simulink library "Feeder1_lib"  (Simulink 8.1)
settings: Solver=ode45  StartTime=0.0  StopTime=10.0  RelTol=1e-3
undefined symbols (not defined in the file): Left, Ts, type, V
libraries: breaker_lib x16, cables_lib x15, transformer_lib x9, Load_lib x6, ssn_lib x6, fault_lib x3, rtlab x2, powerlib x1, HWController_Diesel_GenSet_4MVA_lib x1, Motor_InductionMachine_lib x1, PQFV_lib x1
settings Model: Creator=re25624  LastModifiedBy=RE25624

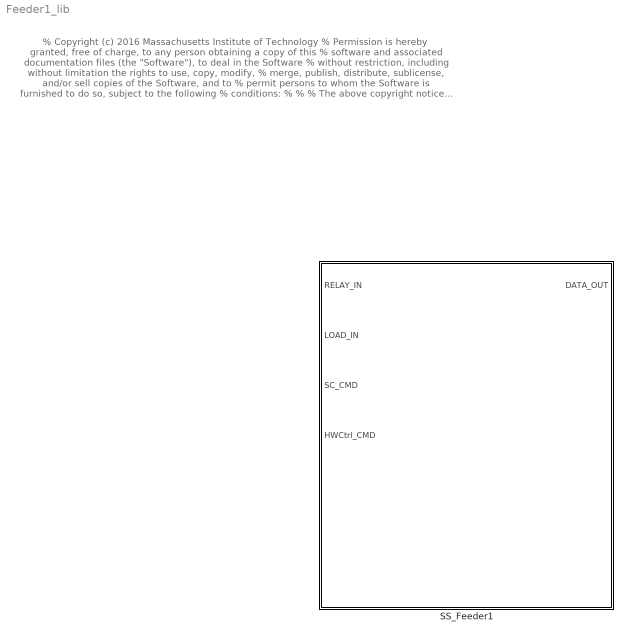
== system Feeder1_lib ==
  note: % Copyright (c) 2016 Massachusetts Institute of Technology
      | % Permission is hereby granted, free of charge, to any person obtaining a copy of this
      | % software and associated documentation files (the "Software"), to deal in the Software
      | % without restriction, including without limitation the rights to use, copy, modify,
      | % merge, publish, distribute, sublicense, and/or sell copies of the Software, and to
      | % permit persons to whom the Software is furnished to do so, subject to the following
      | % conditions:
      | %
      | %
      | % The above copyright notice and this permission notice shall be included in
      | % all copies or substantial portions of the Software.
      | %
      | % THE SOFTWARE IS PROVIDED "AS IS", WITHOUT WARRANTY OF ANY KIND, EXPRESS OR IMPLIED,
      | % INCLUDING BUT NOT LIMITED TO THE WARRANTIES OF MERCHANTABILITY, FITNESS FOR A
      | % PARTICULAR PURPOSE AND NONINFRINGEMENT. IN NO EVENT SHALL THE AUTHORS OR COPYRIGHT
      | % HOLDERS BE LIABLE FOR ANY CLAIM, DAMAGES OR OTHER LIABILITY, WHETHER IN AN ACTION
      | % OF CONTRACT, TORT OR OTHERWISE, ARISING FROM, OUT OF OR IN CONNECTION WITH THE
      | % SOFTWARE OR THE USE OR OTHER DEALINGS IN THE SOFTWARE.
      | %
      | %
      | %%
  SS_Feeder1 : Subsystem

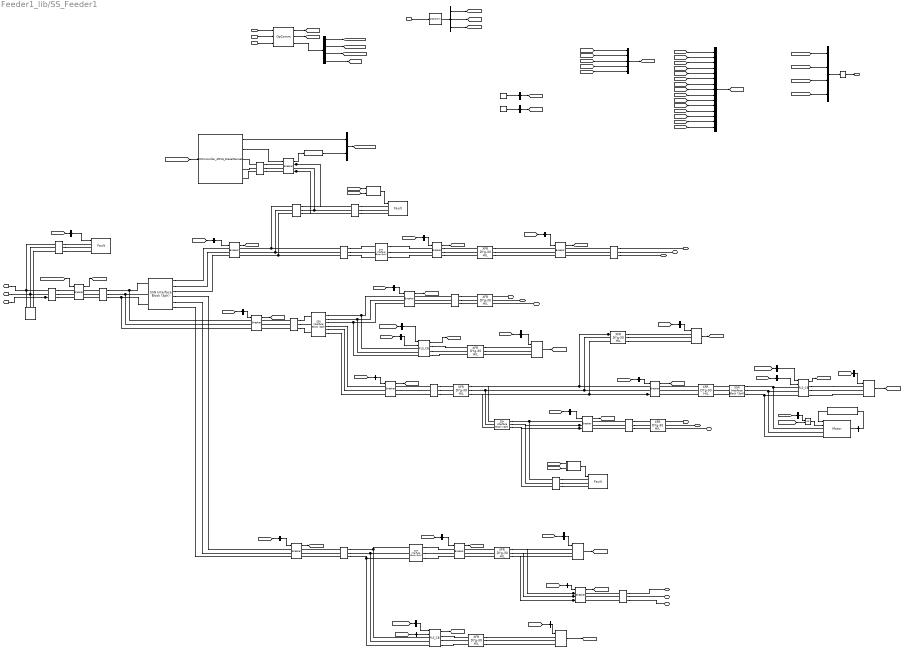
== system Feeder1_lib/SS_Feeder1 ==
  note: % Copyright (c) 2016 Massachusetts Institute of Technology
      | % Permission is hereby granted, free of charge, to any person obtaining a copy of this
      | % software and associated documentation files (the "Software"), to deal in the Software
      | % without restriction, including without limitation the rights to use, copy, modify,
      | % merge, publish, distribute, sublicense, and/or sell copies of the Software, and to
      | % permit persons to whom the Software is furnished to do so, subject to the following
      | % conditions:
      | %
      | %
      | % The above copyright notice and this permission notice shall be included in
      | % all copies or substantial portions of the Software.
      | %
      | % THE SOFTWARE IS PROVIDED "AS IS", WITHOUT WARRANTY OF ANY KIND, EXPRESS OR IMPLIED,
      | % INCLUDING BUT NOT LIMITED TO THE WARRANTIES OF MERCHANTABILITY, FITNESS FOR A
      | % PARTICULAR PURPOSE AND NONINFRINGEMENT. IN NO EVENT SHALL THE AUTHORS OR COPYRIGHT
      | % HOLDERS BE LIABLE FOR ANY CLAIM, DAMAGES OR OTHER LIABILITY, WHETHER IN AN ACTION
      | % OF CONTRACT, TORT OR OTHERWISE, ARISING FROM, OUT OF OR IN CONNECTION WITH THE
      | % SOFTWARE OR THE USE OR OTHER DEALINGS IN THE SOFTWARE.
      | %
      | %
      | %%
  note: connect to F3
  note: connect to F2
  note: connect to F2
  note: connect to F2
  RELAY_IN : Inport
  LOAD_IN : Inport  Port=2
  SC_CMD : Inport  Port=3
  HWCtrl_CMD : Inport  Port=4
  200 HP chiller compressor : Load_lib/200 HP chiller compressor
  2000 kVA4 : transformer_lib/XFR DYg-30 HIL  Rating=2000  Vp=4160  Vs=480  Z=5.75  XR=5.7
  2000 kVA5 : transformer_lib/XFR DYg-30 HIL  Rating=2000  Vp=4160  Vs=480  Z=5.75  XR=5.7
  2500 kVA : transformer_lib/XFR DYg-30 HIL  Rating=2500  Vp=13800  Vs=480  Z=5.75  XR=6.6
  2500 kVA2 : transformer_lib/XFR DYg-30 HIL  Rating=2500  Vp=13800  Vs=480  Z=5.56  XR=5.52
  3750 kVA1 : transformer_lib/XFR DYg-30 HIL  Rating=3750  Vp=13800  Vs=4160  Z=4.75  XR=11.4
  4/0AWG-Mutual1 : cables_lib/4//0AWG-Mutual  length=100  par_sets=1  ratio=3
  448 kvar inductor at 13.8kV  to cancel kvar produced by the stublines1 : powerlib/Elements/Three-Phase Parallel RLC Load  LConnTagsString=A|B|C  Configuration=Y (grounded)  NominalVoltage=13800  NominalFrequency=60  ActivePower=0  InductivePower=448e3  CapacitivePower=0  Measurements=None  LoadType=constant Z
  500 kVA2 : transformer_lib/XFR DYg-30 HIL  Rating=500  Vp=13800  Vs=480  Z=5  XR=4.9
  500 kVA3 : transformer_lib/XFR DYg-30 HIL  Rating=500  Vp=13800  Vs=208  Z=5  XR=4.9
  500kcmil-Mutual1 : cables_lib/500kcmil-Mutual  length=1000  par_sets=1  ratio=3
  500kcmil-Mutual2 : cables_lib/500kcmil-Mutual  length=10  par_sets=1  ratio=3
  500kcmil-Mutual3 : cables_lib/500kcmil-Mutual  length=10  par_sets=1  ratio=3
  500kcmil-Mutual4 : cables_lib/500kcmil-Mutual  length=10  par_sets=1  ratio=3
  500kcmil-Mutual9 : cables_lib/500kcmil-Mutual  length=100  par_sets=1  ratio=3
  Bus Creator : BusCreator  Inputs=1
  Bus Creator1 : BusCreator  Inputs=1
  Bus Creator2 : BusCreator
  Bus Creator3 : BusCreator  Inputs=5
  Bus Creator5 : BusCreator  Inputs=15
  Bus Creator6 : BusCreator  Inputs=2
  Bus Selector : BusSelector  OutputSignals=motor_1
  Bus Selector1 : BusSelector  OutputSignals=F1_CB_12
  Bus Selector10 : BusSelector  OutputSignals=F1_CB_2
  Bus Selector11 : BusSelector  OutputSignals=F1_CB_1
  Bus Selector12 : BusSelector  OutputSignals=F1_CB_5
  Bus Selector13 : BusSelector  OutputSignals=F1_CB_3
  Bus Selector14 : BusSelector  OutputSignals=F1_CB_6
  Bus Selector15 : BusSelector  OutputSignals=F1_CB_7
  Bus Selector16 : BusSelector  OutputSignals=F1_CB_10
  Bus Selector17 : BusSelector  OutputSignals=F1_CB_11
  Bus Selector18 : BusSelector  OutputSignals=F1_CB_9
  Bus Selector19 : BusSelector  OutputSignals=F1_CB_14
  Bus Selector2 : BusSelector  OutputSignals=F1_CB_4
  Bus Selector20 : BusSelector  OutputSignals=fault_cmd,motor_ONOFF.F1_motor_ONOFF,GridStatusCtrl.Grid_F1.Logic_trip
  Bus Selector21 : BusSelector  OutputSignals=HWCtrl.Diesel_Gen2,HWCtrl.SEL751_LogicTrip.F1.Logic_trip,HWCtrl.SEL2440_FLS,TestSeq
  Bus Selector22 : BusSelector  OutputSignals=RPM
  Bus Selector23 : BusSelector  OutputSignals=CB107
  Bus Selector24 : BusSelector  OutputSignals=CB104
  Bus Selector25 : BusSelector  OutputSignals=CB114
  Bus Selector26 : BusSelector  OutputSignals=fault_location_6
  Bus Selector3 : BusSelector  OutputSignals=I2
  Bus Selector4 : BusSelector  OutputSignals=C2
  Bus Selector5 : BusSelector  OutputSignals=P1
  Bus Selector6 : BusSelector  OutputSignals=C1
  Bus Selector7 : BusSelector  OutputSignals=I1
  Bus Selector8 : BusSelector  OutputSignals=F1_CB_13
  Bus Selector9 : BusSelector  OutputSignals=F1_CB_8
  C1 : cables_lib/500kcmil-Mutual  length=10  par_sets=1  ratio=3
  C101 : cables_lib/500kcmil-Mutual  length=1800  par_sets=1  ratio=3
  C102 : cables_lib/500kcmil-Mutual  length=5500  par_sets=1  ratio=3
  C103 : cables_lib/4//0AWG-Mutual  length=1000  par_sets=1  ratio=3
  C104 : cables_lib/500kcmil-Mutual  length=3000  par_sets=1  ratio=3
  C106 : cables_lib/500kcmil-Mutual  length=1500  par_sets=1  ratio=3
  C108 : cables_lib/500kcmil-Mutual  length=10  par_sets=1  ratio=3
  C109 : cables_lib/500kcmil-Mutual  length=1  par_sets=1  ratio=3
  C2 : cables_lib/500kcmil-Mutual  length=10  par_sets=1  ratio=3
  CB closed : Constant
  CB open : Constant  Value=0
  Critical_1 : Load_lib/Dynamic_Load  V=480  kVA=1200  PF=0.9  Ts=Ts
  Critical_2 : Load_lib/Dynamic_Load  V=480  kVA=1500  PF=0.9  Ts=Ts
  F1-GCB : breaker_lib/Breaker  Ts=Ts  mech_delay=cb_mech_delay
  F1_CB_{1..3,5..6,8..13} (11 alike) : breaker_lib/Breaker  Ts=Ts  mech_delay=cb_mech_delay
  F1_CB_14 : breaker_lib/FLS_CB  Ts=Ts  mech_delay=cb_mech_delay
  F1_CB_4 : breaker_lib/FLS_CB  Ts=Ts  mech_delay=cb_mech_delay
  F1_CB_7 : breaker_lib/FLS_CB  Ts=Ts  mech_delay=cb_mech_delay
  F1_PCC : breaker_lib/Breaker  Ts=Ts  mech_delay=cb_mech_delay
  Fault_2 : fault_lib/Fault  FaultResistance=0.1  GroundResistance=1.73  SnubberResistance=1E6
  Fault_3 : fault_lib/Fault  FaultResistance=0.1  GroundResistance=1.73  SnubberResistance=1E6
  Fault_6 : fault_lib/Fault  FaultResistance=0.1  GroundResistance=0.01  SnubberResistance=1E6
  HWController_4MVA_DieselGenset : HWController_Diesel_GenSet_4MVA_lib/HWController_4MVA_DieselGenset
  Interruptible_1 : Load_lib/Dynamic_Load  V=480  kVA=300  PF=0.9  Ts=Ts
  Interruptible_2 : Load_lib/Dynamic_Load  V=208  kVA=250  PF=0.9  Ts=Ts
  Logical Operator : Logic  Operator=OR  AllPortsSameDT=off  OutDataTypeStr=boolean
  Low imp xfr to handle stubline : transformer_lib/XFR DYg-30 HIL  Rating=5000  Vp=13800  Vs=500  Z=0.1  XR=10
  Low imp xfr to handle stubline1 : transformer_lib/XFR DYg-30 HIL  Rating=5000  Vp=4160  Vs=500  Z=0.1  XR=10
  Memory : Memory
  Motor : Motor_InductionMachine_lib/Motor
  OpComm1 : rtlab/OpComm  nbport=3  groupe_acq=1  subsys_rate=0  st=0  Synchronization=on  Interpolation=on  Threshold=1.0  Missed_Data=off  Sim_Time=off  Samples=off  dynSigOut=off  from_console=0  warning_done=off  writeOpCommFile=off  Offset=off
  OpComm2 : rtlab/OpComm  nbport=1  groupe_acq=1  subsys_rate=0  st=0  Synchronization=on  Interpolation=on  Threshold=1.0  Missed_Data=off  Sim_Time=off  Samples=off  dynSigOut=off  from_console=1  warning_done=off  writeOpCommFile=off  Offset=off
  PQFV : PQFV_lib/PQFV  VRMSLL=13800  Ts=Ts
  Priority_1 : Load_lib/Dynamic_Load  V=480  kVA=1000  PF=0.9  Ts=Ts
  SSN Interface Block (3ph) : ssn_lib/SSN Interface Block (3ph)  nb_phase=3  nb_port=3  p1_type=V-type(Left)  p2_type=V-type (Right)  p3_type=V-type (Right)  p4_type=V-type (Right)  p5_type=V-type(Left)  p6_type=V-type(Left)  p7_type=V-type(Left)  p8_type=V-type(Left)  p9_type=V-type(Left)  p10_type=V-type(Left)  p11_type=V-type(Left)  p12_type=V-type(Left)  p13_type=V-type(Left)  p14_type=V-type(Left)  p15_type=V-type(Left)  p16_type=V-type(Left)  I_port_shunt_resistance=1e9
  SSN Interface Block (3ph)1 : ssn_lib/SSN Interface Block (3ph)  nb_phase=3  nb_port=3  p1_type=V-type(Left)  p2_type=V-type (Right)  p3_type=V-type (Right)  p4_type=V-type(Left)  p5_type=V-type(Left)  p6_type=V-type(Left)  p7_type=V-type(Left)  p8_type=V-type(Left)  p9_type=V-type(Left)  p10_type=V-type(Left)  p11_type=V-type(Left)  p12_type=V-type(Left)  p13_type=V-type(Left)  p14_type=V-type(Left)  p15_type=V-type(Left)  p16_type=V-type(Left)  I_port_shunt_resistance=1e9
  SSN Interface Block (3ph){2..4,12} (4 alike) : ssn_lib/SSN Interface Block (3ph)  nb_phase=3  nb_port=2  p1_type=V-type(Left)  p2_type=V-type (Right)  p3_type=V-type(Left)  p4_type=V-type(Left)  p5_type=V-type(Left)  p6_type=V-type(Left)  p7_type=V-type(Left)  p8_type=V-type(Left)  p9_type=V-type(Left)  p10_type=V-type(Left)  p11_type=V-type(Left)  p12_type=V-type(Left)  p13_type=V-type(Left)  p14_type=V-type(Left)  p15_type=V-type(Left)  p16_type=V-type(Left)  I_port_shunt_resistance=1e9
  fault_signal : Subsystem
  fault_signal1 : Subsystem
  A_CB_8 : PMIOPort  Port=1  Side=Right
  B_CB_8 : PMIOPort  Port=2  Side=Right
  C_CB_8 : PMIOPort  Port=3  Side=Right
  A_CB_11 : PMIOPort  Port=4  Side=Right
  B_CB_11 : PMIOPort  Port=5  Side=Right
  C_CB_11 : PMIOPort  Port=6  Side=Right
  A_CB_9 : PMIOPort  Port=7  Side=Right
  B_CB_9 : PMIOPort  Port=8  Side=Right
  C_CB_9 : PMIOPort  Port=9  Side=Right
  A_CB_13 : PMIOPort  Port=10  Side=Right
  B_CB_13 : PMIOPort  Port=11  Side=Right
  C_CB_13 : PMIOPort  Port=12  Side=Right
  PCC_A : PMIOPort  Port=13  Side=Left
  PCC_B : PMIOPort  Port=14  Side=Left
  PCC_C : PMIOPort  Port=15  Side=Left
  DATA_OUT : Outport
  wires:
  Bus Selector26/1 -> Fault_6/1  "<fault_location_6>"
  [fault_cmd] -> Bus Selector26/1
  fault_signal/1(o) -> Fault_2/1
  Logical Operator/1 -> Motor/2
  [motor_cmd] -> Logical Operator/2
  Bus Selector/1 -> Logical Operator/1  "<motor_1>"
  [TestSeq] -> Bus Selector/1
  fault_signal1/1(o) -> Fault_3/1
  [fault_cmd] -> fault_signal1/2(fault_sc)
  [TestSeq] -> fault_signal1/1(fault_ts)
  [fault_cmd] -> fault_signal/2(fault_sc)
  [TestSeq] -> fault_signal/1(fault_ts)
  Bus Selector21/4 -> [TestSeq]  "<TestSeq>"
  Bus Selector20/3 -> [feeder_cb]  "<Logic_trip>"
  Bus Selector25/1 -> F1_CB_14/1  "<CB114>"
  [SEL_2440_FLS] -> Bus Selector25/1
  Bus Selector24/1 -> F1_CB_4/1  "<CB104>"
  [SEL_2440_FLS] -> Bus Selector24/1
  Bus Selector21/3 -> [SEL_2440_FLS]  "<SEL2440_FLS>"
  Bus Selector23/1 -> F1_CB_7/1  "<CB107>"
  [SEL_2440_FLS] -> Bus Selector23/1
  [SEL751_F1_LogicTrip] -> F1_PCC/1
  Bus Selector21/2 -> [SEL751_F1_LogicTrip]  "<Logic_trip>"
  [motor_cmd] -> Bus Creator2/4  "MOTOR_ONOFF"
  Bus Selector20/2 -> [motor_cmd]  "<F1_motor_ONOFF>"
  200 HP chiller compressor/1 -> Motor/1
  Bus Selector22/1 -> 200 HP chiller compressor/1  "<RPM>"
  Motor/1 -> Bus Selector22/1
  [DIESEL_DATA] -> Bus Creator2/3  "DIESEL_DATA"
  [LOAD_DATA] -> Bus Creator2/2  "LOAD_DATA"
  [CB_DATA] -> Bus Creator2/1  "CB_DATA"
  Bus Creator2/1 -> Memory/1
  Memory/1 -> DATA_OUT/1
  HWController_4MVA_DieselGenset/1 -> Bus Creator6/1  "Gen2_meas"
  PQFV/1 -> Bus Creator6/2  "DIESEL_GCB"
  Bus Creator6/1 -> [DIESEL_DATA]
  F1-GCB/1 -> PQFV/1
  HWCtrl_CMD/1 -> OpComm1/3
  Bus Selector21/1 -> [Diesel_Gen2]  "<Diesel_Gen2>"
  OpComm1/3 -> Bus Selector21/1
  HWController_4MVA_DieselGenset/2 -> F1-GCB/1
  [Diesel_Gen2] -> HWController_4MVA_DieselGenset/1
  Bus Creator5/1 -> [CB_DATA]
  Bus Creator3/1 -> [LOAD_DATA]  "LOAD"
  Bus Selector20/1 -> [fault_cmd]  "<fault_cmd>"
  OpComm2/1 -> Bus Selector20/1
  SC_CMD/1 -> OpComm2/1
  [F1_CB_14] -> Bus Creator5/14  "F1_CB_14"
  [F1_PCC] -> Bus Creator5/15  "F1_PCC"
  Bus Selector19/1 -> F1_CB_14/2  "<F1_CB_14>"
  [RELAY_IN] -> Bus Selector19/1
  F1_CB_14/1 -> [F1_CB_14]
  Bus Selector2/1 -> F1_CB_4/2  "<F1_CB_4>"
  [RELAY_IN] -> Bus Selector2/1
  F1_CB_4/1 -> [F1_CB_4]
  F1_CB_2/1 -> [F1_CB_2]
  Bus Selector18/1 -> F1_CB_9/1  "<F1_CB_9>"
  Bus Selector12/1 -> F1_CB_5/1  "<F1_CB_5>"
  Bus Selector11/1 -> F1_CB_1/1  "<F1_CB_1>"
  Bus Selector17/1 -> F1_CB_11/1  "<F1_CB_11>"
  Bus Selector16/1 -> F1_CB_10/1  "<F1_CB_10>"
  Bus Selector10/1 -> F1_CB_2/1  "<F1_CB_2>"
  Bus Selector14/1 -> F1_CB_6/1  "<F1_CB_6>"
  Bus Selector15/1 -> F1_CB_7/2  "<F1_CB_7>"
  Bus Selector9/1 -> F1_CB_8/1  "<F1_CB_8>"
  Bus Selector8/1 -> F1_CB_13/1  "<F1_CB_13>"
  Bus Selector1/1 -> F1_CB_12/1  "<F1_CB_12>"
  [RELAY_IN] -> Bus Selector18/1
  [RELAY_IN] -> Bus Selector17/1
  [RELAY_IN] -> Bus Selector16/1
  [RELAY_IN] -> Bus Selector15/1
  [RELAY_IN] -> Bus Selector14/1
  [RELAY_IN] -> Bus Selector12/1
  [RELAY_IN] -> Bus Selector11/1
  [RELAY_IN] -> Bus Selector10/1
  [RELAY_IN] -> Bus Selector9/1
  [RELAY_IN] -> Bus Selector8/1
  [RELAY_IN] -> Bus Selector1/1
  [RELAY_IN] -> Bus Selector13/1
  Bus Selector13/1 -> F1_CB_3/1  "<F1_CB_3>"
  OpComm1/2 -> [RELAY_IN]
  RELAY_IN/1 -> OpComm1/2
  [F1_CB_2] -> Bus Creator5/2  "F1_CB_2"
  [F1_CB_3] -> Bus Creator5/3  "F1_CB_3"
  [F1_CB_4] -> Bus Creator5/4  "F1_CB_4"
  [F1_CB_5] -> Bus Creator5/5  "F1_CB_5"
  [F1_CB_6] -> Bus Creator5/6  "F1_CB_6"
  [F1_CB_7] -> Bus Creator5/7  "F1_CB_7"
  [F1_CB_8] -> Bus Creator5/8  "F1_CB_8"
  [F1_CB_9] -> Bus Creator5/9  "F1_CB_9"
  [F1_CB_10] -> Bus Creator5/10  "F1_CB_10"
  [F1_CB_11] -> Bus Creator5/11  "F1_CB_11"
  [F1_CB_12] -> Bus Creator5/12  "F1_CB_12"
  [F1_CB_13] -> Bus Creator5/13  "F1_CB_13"
  [F1_CB_1] -> Bus Creator5/1  "F1_CB_1"
  F1_CB_11/1 -> [F1_CB_11]
  F1_CB_10/1 -> [F1_CB_10]
  F1_CB_13/1 -> [F1_CB_13]
  F1_CB_12/1 -> [F1_CB_12]
  F1_CB_8/1 -> [F1_CB_8]
  F1_CB_7/1 -> [F1_CB_7]
  F1_CB_6/1 -> [F1_CB_6]
  F1_CB_9/1 -> [F1_CB_9]
  F1_CB_5/1 -> [F1_CB_5]
  F1_CB_1/1 -> [F1_CB_1]
  F1_CB_3/1 -> [F1_CB_3]
  [LOAD_I1] -> Bus Creator3/3  "F1_I1"
  [LOAD_C2] -> Bus Creator3/2  "F1_C2"
  [LOAD_P1] -> Bus Creator3/5  "F1_P1"
  [LOAD_I2] -> Bus Creator3/4  "F1_I2"
  [LOAD_C1] -> Bus Creator3/1  "F1_C1"
  Interruptible_1/1 -> [LOAD_I1]
  Critical_1/1 -> [LOAD_C1]
  Priority_1/1 -> [LOAD_P1]
  Critical_2/1 -> [LOAD_C2]
  Interruptible_2/1 -> [LOAD_I2]
  Bus Selector7/1 -> Interruptible_1/1  "<I1>"
  Bus Selector6/1 -> Critical_1/1  "<C1>"
  Bus Selector5/1 -> Priority_1/1  "<P1>"
  Bus Selector4/1 -> Critical_2/1  "<C2>"
  Bus Selector3/1 -> Interruptible_2/1  "<I2>"
  [LOAD_IN] -> Bus Selector7/1
  [LOAD_IN] -> Bus Selector6/1
  [LOAD_IN] -> Bus Selector5/1
  [LOAD_IN] -> Bus Selector4/1
  [LOAD_IN] -> Bus Selector3/1
  OpComm1/1 -> [LOAD_IN]
  LOAD_IN/1 -> OpComm1/1
  CB open/1 -> Bus Creator1/1  "Logic_trip"
  Bus Creator1/1 -> [cb_o]
  CB closed/1 -> Bus Creator/1  "Logic_trip"
  Bus Creator/1 -> [cb_c]
  F1_PCC/1 -> [F1_PCC]
  connections:
  500kcmil-Mutual4/RConn1 -- Fault_6/LConn1
  500kcmil-Mutual4/RConn3 -- Fault_6/LConn3
  500kcmil-Mutual4/RConn2 -- Fault_6/LConn2
  C2/LConn2 -- F1_CB_8/RConn2
  C2/LConn1 -- F1_CB_8/RConn1
  C2/LConn3 -- F1_CB_8/RConn3
  C2/RConn3 -- Low imp xfr to handle stubline/LConn3
  C2/RConn1 -- Low imp xfr to handle stubline/LConn1
  C2/RConn2 -- Low imp xfr to handle stubline/LConn2
  C1/LConn1 -- F1_CB_11/RConn1
  C1/LConn2 -- F1_CB_11/RConn2
  C1/LConn3 -- F1_CB_11/RConn3
  C_CB_11/RConn1 -- Low imp xfr to handle stubline1/RConn3
  B_CB_11/RConn1 -- Low imp xfr to handle stubline1/RConn2
  A_CB_11/RConn1 -- Low imp xfr to handle stubline1/RConn1
  C1/RConn3 -- Low imp xfr to handle stubline1/LConn3
  C1/RConn2 -- Low imp xfr to handle stubline1/LConn2
  C1/RConn1 -- Low imp xfr to handle stubline1/LConn1
  C_CB_8/RConn1 -- Low imp xfr to handle stubline/RConn3
  B_CB_8/RConn1 -- Low imp xfr to handle stubline/RConn2
  A_CB_8/RConn1 -- Low imp xfr to handle stubline/RConn1
  500kcmil-Mutual2/RConn1 -- Fault_3/LConn1
  500kcmil-Mutual2/RConn3 -- Fault_3/LConn3
  500kcmil-Mutual2/RConn2 -- Fault_3/LConn2
  500kcmil-Mutual3/RConn1 -- Fault_2/LConn1
  500kcmil-Mutual3/RConn3 -- Fault_2/LConn3
  500kcmil-Mutual3/RConn2 -- Fault_2/LConn2
  448 kvar inductor at 13.8kV  to cancel kvar produced by the stublines1/LConn1 -- 500kcmil-Mutual1/LConn1 -- 500kcmil-Mutual4/LConn1 -- PCC_A/RConn1
  500kcmil-Mutual1/LConn3 -- 448 kvar inductor at 13.8kV  to cancel kvar produced by the stublines1/LConn3 -- 500kcmil-Mutual4/LConn3 -- PCC_C/RConn1
  448 kvar inductor at 13.8kV  to cancel kvar produced by the stublines1/LConn2 -- 500kcmil-Mutual1/LConn2 -- 500kcmil-Mutual4/LConn2 -- PCC_B/RConn1
  F1_CB_2/LConn1 -- SSN Interface Block (3ph)/LConn1 -- 500kcmil-Mutual9/RConn1
  F1_CB_2/LConn3 -- SSN Interface Block (3ph)/LConn3 -- 500kcmil-Mutual9/RConn3
  F1_CB_2/LConn2 -- SSN Interface Block (3ph)/LConn2 -- 500kcmil-Mutual9/RConn2
  500kcmil-Mutual1/RConn1 -- F1_PCC/LConn1
  500kcmil-Mutual1/RConn2 -- F1_PCC/LConn2
  500kcmil-Mutual1/RConn3 -- F1_PCC/LConn3
  500kcmil-Mutual9/LConn3 -- F1_PCC/RConn3
  500kcmil-Mutual9/LConn1 -- F1_PCC/RConn1
  500kcmil-Mutual9/LConn2 -- F1_PCC/RConn2
  C108/RConn3 -- C_CB_9/RConn1
  C108/RConn1 -- A_CB_9/RConn1
  C108/RConn2 -- B_CB_9/RConn1
  C109/RConn1 -- A_CB_13/RConn1
  C109/RConn2 -- B_CB_13/RConn1
  C109/RConn3 -- C_CB_13/RConn1
  4/0AWG-Mutual1/LConn3 -- HWController_4MVA_DieselGenset/RConn3
  4/0AWG-Mutual1/LConn2 -- HWController_4MVA_DieselGenset/RConn2
  4/0AWG-Mutual1/LConn1 -- HWController_4MVA_DieselGenset/RConn1
  4/0AWG-Mutual1/RConn2 -- F1-GCB/LConn2
  4/0AWG-Mutual1/RConn1 -- F1-GCB/LConn1
  4/0AWG-Mutual1/RConn3 -- F1-GCB/LConn3
  500 kVA2/RConn1 -- Interruptible_1/LConn1
  500 kVA2/RConn2 -- Interruptible_1/LConn2
  500 kVA2/RConn3 -- Interruptible_1/LConn3
  SSN Interface Block (3ph)4/LConn1 -- 2000 kVA5/RConn1
  SSN Interface Block (3ph)4/LConn2 -- 2000 kVA5/RConn2
  SSN Interface Block (3ph)4/LConn3 -- 2000 kVA5/RConn3
  2000 kVA4/RConn2 -- Critical_2/LConn2
  2000 kVA4/RConn1 -- Critical_2/LConn1
  2000 kVA4/RConn3 -- Critical_2/LConn3
  500 kVA3/RConn1 -- Interruptible_2/LConn1
  500 kVA3/RConn2 -- Interruptible_2/LConn2
  500 kVA3/RConn3 -- Interruptible_2/LConn3
  F1-GCB/RConn1 -- 500kcmil-Mutual3/LConn1 -- C103/RConn1
  500kcmil-Mutual3/LConn2 -- F1-GCB/RConn2 -- C103/RConn2
  F1-GCB/RConn3 -- 500kcmil-Mutual3/LConn3 -- C103/RConn3
  F1_CB_14/LConn1 -- Motor/LConn1 -- SSN Interface Block (3ph)4/RConn1
  F1_CB_14/LConn3 -- Motor/LConn3 -- SSN Interface Block (3ph)4/RConn3
  F1_CB_14/LConn2 -- Motor/LConn2 -- SSN Interface Block (3ph)4/RConn2
  C106/RConn1 -- 3750 kVA1/LConn1
  C106/RConn3 -- 3750 kVA1/LConn3
  C106/RConn2 -- 3750 kVA1/LConn2
  SSN Interface Block (3ph)1/RConn5 -- F1_CB_6/LConn2
  SSN Interface Block (3ph)1/RConn4 -- F1_CB_6/LConn1
  SSN Interface Block (3ph)1/RConn6 -- F1_CB_6/LConn3
  SSN Interface Block (3ph)1/RConn3 -- F1_CB_7/LConn3 -- F1_CB_8/LConn3
  SSN Interface Block (3ph)1/RConn2 -- F1_CB_7/LConn2 -- F1_CB_8/LConn2
  SSN Interface Block (3ph)1/RConn1 -- F1_CB_7/LConn1 -- F1_CB_8/LConn1
  2000 kVA4/LConn1 -- 3750 kVA1/RConn1 -- SSN Interface Block (3ph)12/LConn1 -- F1_CB_10/LConn1
  F1_CB_11/LConn2 -- 500kcmil-Mutual2/LConn2 -- SSN Interface Block (3ph)12/RConn2
  F1_CB_10/LConn3 -- 3750 kVA1/RConn3 -- SSN Interface Block (3ph)12/LConn3 -- 2000 kVA4/LConn3
  SSN Interface Block (3ph)3/RConn3 -- F1_CB_12/LConn3
  SSN Interface Block (3ph)3/RConn1 -- F1_CB_12/LConn1
  SSN Interface Block (3ph)3/RConn2 -- F1_CB_12/LConn2
  C104/RConn1 -- SSN Interface Block (3ph)3/LConn1
  C104/RConn3 -- SSN Interface Block (3ph)3/LConn3
  C104/RConn2 -- SSN Interface Block (3ph)3/LConn2
  C109/LConn2 -- F1_CB_13/RConn2
  C109/LConn3 -- F1_CB_13/RConn3
  C109/LConn1 -- F1_CB_13/RConn1
  SSN Interface Block (3ph)/RConn3 -- F1_CB_3/LConn3
  SSN Interface Block (3ph)/RConn2 -- F1_CB_3/LConn2
  SSN Interface Block (3ph)/RConn1 -- F1_CB_3/LConn1
  SSN Interface Block (3ph)2/RConn3 -- F1_CB_5/LConn3
  SSN Interface Block (3ph)2/RConn1 -- F1_CB_5/LConn1
  SSN Interface Block (3ph)2/RConn2 -- F1_CB_5/LConn2
  F1_CB_14/RConn3 -- Priority_1/LConn3
  F1_CB_14/RConn2 -- Priority_1/LConn2
  F1_CB_14/RConn1 -- Priority_1/LConn1
  F1_CB_4/RConn2 -- 500 kVA2/LConn2
  F1_CB_4/RConn3 -- 500 kVA2/LConn3
  F1_CB_4/RConn1 -- 500 kVA2/LConn1
  SSN Interface Block (3ph)12/RConn1 -- 500kcmil-Mutual2/LConn1 -- F1_CB_11/LConn1
  3750 kVA1/RConn2 -- SSN Interface Block (3ph)12/LConn2 -- F1_CB_10/LConn2 -- 2000 kVA4/LConn2
  F1_CB_11/LConn3 -- 500kcmil-Mutual2/LConn3 -- SSN Interface Block (3ph)12/RConn3
  F1_CB_9/LConn3 -- Critical_1/LConn3 -- 2500 kVA2/RConn3
  SSN Interface Block (3ph)2/LConn1 -- F1_CB_4/LConn1 -- C101/RConn1
  2500 kVA/RConn3 -- F1_CB_13/LConn3
  SSN Interface Block (3ph)2/LConn2 -- F1_CB_4/LConn2 -- C101/RConn2
  F1_CB_7/RConn2 -- 500 kVA3/LConn2
  F1_CB_7/RConn1 -- 500 kVA3/LConn1
  2500 kVA/RConn1 -- F1_CB_13/LConn1
  C108/LConn3 -- F1_CB_9/RConn3
  C103/LConn3 -- C104/LConn3 -- F1_CB_3/RConn3
  C101/LConn3 -- F1_CB_1/RConn3
  C108/LConn2 -- F1_CB_9/RConn2
  C108/LConn1 -- F1_CB_9/RConn1
  C103/LConn1 -- C104/LConn1 -- F1_CB_3/RConn1
  2000 kVA5/LConn3 -- F1_CB_10/RConn3
  C101/LConn2 -- F1_CB_1/RConn2
  F1_CB_7/RConn3 -- 500 kVA3/LConn3
  F1_CB_12/RConn3 -- 2500 kVA/LConn3
  C101/LConn1 -- F1_CB_1/RConn1
  F1_CB_12/RConn2 -- 2500 kVA/LConn2
  2000 kVA5/LConn2 -- F1_CB_10/RConn2
  C106/LConn3 -- F1_CB_6/RConn3
  C103/LConn2 -- C104/LConn2 -- F1_CB_3/RConn2
  2500 kVA2/LConn1 -- F1_CB_5/RConn1
  2000 kVA5/LConn1 -- F1_CB_10/RConn1
  C106/LConn2 -- F1_CB_6/RConn2
  SSN Interface Block (3ph)/RConn4 -- F1_CB_1/LConn1
  SSN Interface Block (3ph)/RConn5 -- F1_CB_1/LConn2
  SSN Interface Block (3ph)/RConn6 -- F1_CB_1/LConn3
  F1_CB_12/RConn1 -- 2500 kVA/LConn1
  SSN Interface Block (3ph)2/LConn3 -- F1_CB_4/LConn3 -- C101/RConn3
  F1_CB_9/LConn1 -- Critical_1/LConn1 -- 2500 kVA2/RConn1
  C102/LConn1 -- F1_CB_2/RConn1
  C102/LConn3 -- F1_CB_2/RConn3
  2500 kVA2/LConn2 -- F1_CB_5/RConn2
  C102/LConn2 -- F1_CB_2/RConn2
  2500 kVA2/LConn3 -- F1_CB_5/RConn3
  2500 kVA/RConn2 -- F1_CB_13/LConn2
  C106/LConn1 -- F1_CB_6/RConn1
  F1_CB_9/LConn2 -- Critical_1/LConn2 -- 2500 kVA2/RConn2
  C102/RConn2 -- SSN Interface Block (3ph)1/LConn2
  C102/RConn3 -- SSN Interface Block (3ph)1/LConn3
  C102/RConn1 -- SSN Interface Block (3ph)1/LConn1

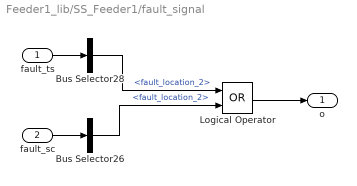
== system Feeder1_lib/SS_Feeder1/fault_signal ==
  fault_ts : Inport
  fault_sc : Inport  Port=2
  Bus Selector26 : BusSelector  OutputSignals=fault_location_2
  Bus Selector28 : BusSelector  OutputSignals=fault_location_2
  Logical Operator : Logic  Operator=OR  AllPortsSameDT=off  OutDataTypeStr=boolean
  o : Outport
  wires:
  Bus Selector28/1 -> Logical Operator/1  "<fault_location_2>"
  Logical Operator/1 -> o/1
  fault_ts/1 -> Bus Selector28/1
  Bus Selector26/1 -> Logical Operator/2  "<fault_location_2>"
  fault_sc/1 -> Bus Selector26/1

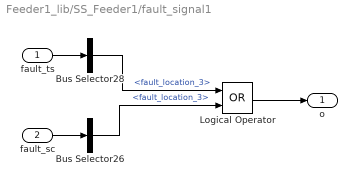
== system Feeder1_lib/SS_Feeder1/fault_signal1 ==
  fault_ts : Inport
  fault_sc : Inport  Port=2
  Bus Selector26 : BusSelector  OutputSignals=fault_location_3
  Bus Selector28 : BusSelector  OutputSignals=fault_location_3
  Logical Operator : Logic  Operator=OR  AllPortsSameDT=off  OutDataTypeStr=boolean
  o : Outport
  wires:
  Bus Selector28/1 -> Logical Operator/1  "<fault_location_3>"
  Logical Operator/1 -> o/1
  fault_ts/1 -> Bus Selector28/1
  Bus Selector26/1 -> Logical Operator/2  "<fault_location_3>"
  fault_sc/1 -> Bus Selector26/1
